simulink model "sampleModel1920"  (R2023a)
settings: Solver=VariableStepAuto  StartTime=0.0  StopTime=10.0  RelTol=1e-3
libraries: hdlsllib x4, simulink x2
settings Model: Creator=user1  LastModifiedBy=user1

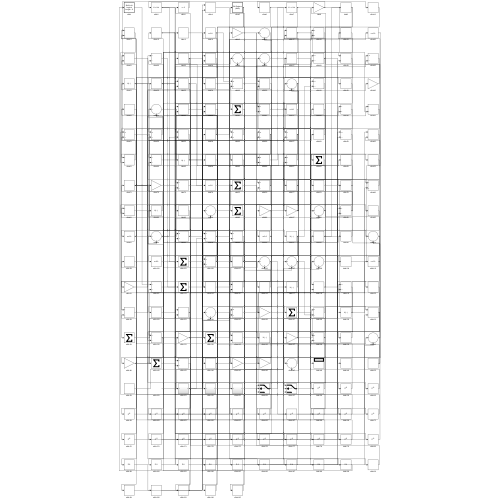
[thumbnail: Simulink's stored preview of the top-level diagram]
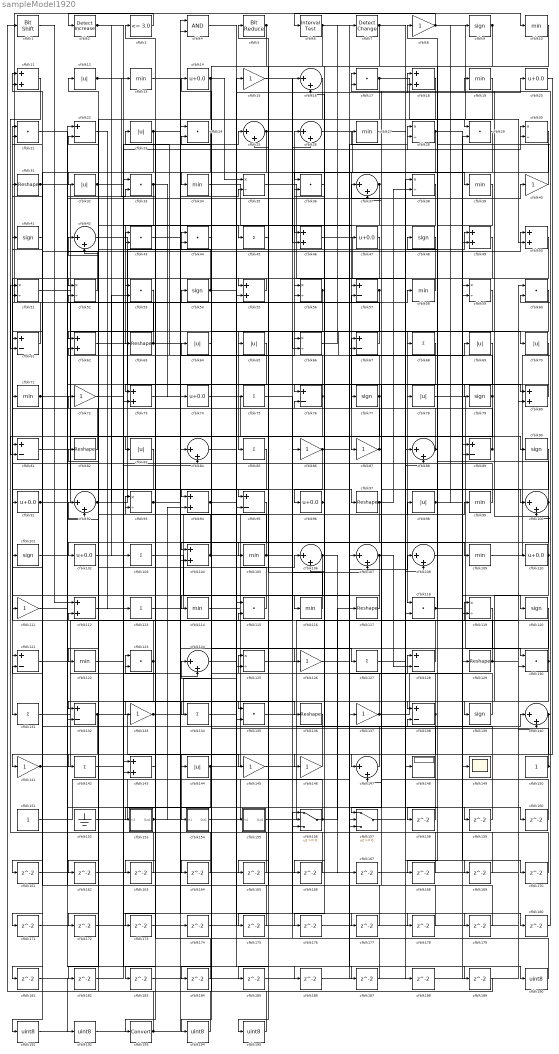
== system sampleModel1920 ==
  cfblk1 : hdlsllib/Logic and Bit Operations/Bit Shift  mode=Shift Left Logical  N=0
  cfblk{10,13,19,27,34,39,58,71,99,105,109,114,116,122} (14 alike) : MinMax
  cfblk{16,25..26,37,42,84,88,92,100,106..108,124,140,147} (15 alike) : Sum  Inputs=|++
  cfblk{9,41,48,54,77,79,90,101,120,139} (10 alike) : Signum
  cfblk{14,20,47,74,91,96,102,110} (8 alike) : Bias  Bias=0.0  SaturateOnIntegerOverflow=off
  cfblk{45,68,75,85,103,113,127,131,134,142} (10 alike) : Sum  Inputs=+
  cfblk{11,18,46,49..50,55,62,73,80,94,104,112,143} (13 alike) : Sum
  cfblk{8,15,40,72,86..87,111,126,133,137,141,145..146} (13 alike) : Gain
  cfblk{17,21,24,29,33,36,43..44,53,60,115,118,123,130,135} (15 alike) : DotProduct  OutDataTypeStr=Inherit: Inherit via internal rule
  cfblk{31,63,82,97,117,129,136} (7 alike) : Reshape
  cfblk{28,30,35,38,51..52,56,59,66,93,119,125} (12 alike) : Product  Inputs=*/  RndMeth=Zero  SaturateOnIntegerOverflow=on
  cfblk{12,23,32,64..65,69..70,78,83,98,144} (11 alike) : Abs  SaturateOnIntegerOverflow=off
  cfblk{22,57,61,67,76,81,89,95,121,128,132,138} (12 alike) : Sum  Inputs=+-
  cfblk148 : Display
  cfblk149 : Scope
  cfblk150 : Constant  SampleTime=-1
  cfblk151 : Constant  SampleTime=-1
  cfblk152 : Ground
  cfblk153 : Subsystem
      settings: LibrarySourceBlock=|
      | hdlsllib/Ports &
      | Subsystems/Subsystem
  cfblk154 : Subsystem
      settings: LibrarySourceBlock=|
      | hdlsllib/Ports &
      | Subsystems/Subsystem
  cfblk155 : Subsystem
      settings: LibrarySourceBlock=|
      | hdlsllib/Ports &
      | Subsystems/Subsystem
  cfblk156 : Switch  SaturateOnIntegerOverflow=off  InputSameDT=off
  cfblk157 : Switch  SaturateOnIntegerOverflow=off  InputSameDT=off
  cfblk{158..189} (32 alike) : Delay  SampleTime=1
  cfblk{190..192,194..195} (5 alike) : DataTypeConversion  OutDataTypeStr=uint8  SaturateOnIntegerOverflow=off  RndMeth=Floor
  cfblk193 : DataTypeConversion  SaturateOnIntegerOverflow=off  RndMeth=Floor
  cfblk2 : simulink/Logic and Bit Operations/Detect Increase  vinit=0.0  OutDataTypeStr=boolean
      settings: LibrarySourceBlock=|
      | hdlsllib/Logic and Bit
      | Operations/Detect
      | Increase
  cfblk3 : hdlsllib/Logic and Bit Operations/Compare To Constant  relop=<=  const=3.0  OutDataTypeStr=boolean
  cfblk4 : Logic  AllPortsSameDT=off  OutDataTypeStr=boolean
  cfblk5 : hdlsllib/Logic and Bit Operations/Bit Reduce  mode=AND
  cfblk6 : hdlsllib/Logic and Bit Operations/Interval Test  IntervalClosedRight=on  uplimit=0.5  IntervalClosedLeft=on  lowlimit=-0.5  OutDataTypeStr=boolean
  cfblk7 : simulink/Logic and Bit Operations/Detect Change  vinit=0  OutDataTypeStr=boolean
      settings: LibrarySourceBlock=|
      | hdlsllib/Logic and Bit
      | Operations/Detect
      | Change
  wires:
  cfblk66/1 -> cfblk7/1
  cfblk86/1 -> cfblk96/1, cfblk28/2
  cfblk1/1 -> cfblk112/1
  cfblk68/1 -> cfblk118/1
  cfblk33/1 -> cfblk74/1, cfblk52/1
  cfblk2/1 -> cfblk103/1, cfblk66/2, cfblk177/1
  cfblk78/1 -> cfblk130/1
  cfblk60/1 -> cfblk23/1
  cfblk136/1 -> cfblk154/1(In1)
  cfblk22/1 -> cfblk113/1
  cfblk56/1 -> cfblk85/1, cfblk135/1
  cfblk109/1 -> cfblk17/1
  cfblk128/1 -> cfblk13/1
  cfblk134/1 -> cfblk15/1
  cfblk20/1 -> cfblk147/1
  cfblk59/1 -> cfblk78/1
  cfblk62/1 -> cfblk49/1
  cfblk42/1 -> cfblk76/1
  cfblk30/1 -> cfblk87/1
  cfblk144/1 -> cfblk106/1, cfblk173/1
  cfblk58/1 -> cfblk57/1
  cfblk150/1 -> cfblk44/1, cfblk100/2
  cfblk153/1(Out1) -> cfblk99/1, cfblk94/2, cfblk57/2
  cfblk113/1 -> cfblk98/1
  cfblk129/1 -> cfblk110/1, cfblk93/1
  cfblk132/1 -> cfblk145/1, cfblk181/1
  cfblk115/1 -> cfblk12/1
  cfblk84/1 -> cfblk109/1
  cfblk92/1 -> cfblk58/1, cfblk53/2
  cfblk61/1 -> cfblk10/1
  cfblk3/1 -> cfblk2/1
  cfblk117/1 -> cfblk116/1
  cfblk12/1 -> cfblk45/1, cfblk97/1
  cfblk45/1 -> cfblk95/1
  cfblk49/1 -> cfblk131/1
  cfblk6/1 -> cfblk79/1, cfblk34/1
  cfblk77/1 -> cfblk26/1, cfblk156/3
  cfblk47/1 -> cfblk55/1
  cfblk87/1 -> cfblk21/1, cfblk27/1, cfblk37/2
  cfblk131/1 -> cfblk123/1
  cfblk155/1(Out1) -> cfblk140/1
  cfblk118/1 -> cfblk18/1, cfblk120/1
  cfblk122/1 -> cfblk25/1
  cfblk106/1 -> cfblk134/1, cfblk167/1
  cfblk46/1 -> cfblk88/1
  cfblk107/1 -> cfblk121/1, cfblk128/2
  cfblk111/1 -> cfblk50/1
  cfblk36/1 -> cfblk106/2
  cfblk91/1 -> cfblk54/1, cfblk11/2
  cfblk141/1 -> cfblk86/1, cfblk66/1
  cfblk31/1 -> cfblk70/1, cfblk186/1
  cfblk93/1 -> cfblk3/1, cfblk28/1
  cfblk96/1 -> cfblk36/2, cfblk166/1
  cfblk24/1 -> cfblk193/1
  cfblk54/1 -> cfblk22/2, cfblk20/1
  cfblk105/1 -> cfblk16/1, cfblk107/2, cfblk82/1, cfblk180/1
  cfblk135/1 -> cfblk38/1
  cfblk76/1 -> cfblk5/1, cfblk94/1, cfblk62/2
  cfblk81/1 -> cfblk90/1
  cfblk146/1 -> cfblk141/1
  cfblk52/1 -> cfblk11/1
  cfblk15/1 -> cfblk47/1
  cfblk37/1 -> cfblk63/1, cfblk157/2
  cfblk102/1 -> cfblk143/1
  cfblk108/1 -> cfblk149/1
  cfblk139/1 -> cfblk44/2
  cfblk55/1 -> cfblk53/1
  cfblk38/1 -> cfblk83/1
  cfblk90/1 -> cfblk147/2
  cfblk123/1 -> cfblk71/1, cfblk132/2
  cfblk14/1 -> cfblk32/1, cfblk35/1
  cfblk48/1 -> cfblk118/2
  cfblk16/1 -> cfblk55/2
  cfblk69/1 -> cfblk157/1
  cfblk156/1 -> cfblk125/1, cfblk117/1
  cfblk17/1 -> cfblk29/1, cfblk62/1
  cfblk140/1 -> cfblk60/2, cfblk191/1
  cfblk99/1 -> cfblk81/1
  cfblk43/1 -> cfblk127/1
  cfblk18/1 -> cfblk102/1
  cfblk10/1 -> cfblk68/1
  cfblk94/1 -> cfblk18/2, cfblk184/1
  cfblk114/1 -> cfblk49/2
  cfblk152/1 -> cfblk128/1
  cfblk80/1 -> cfblk73/1
  cfblk137/1 -> cfblk59/1, cfblk43/1
  cfblk95/1 -> cfblk122/1
  cfblk138/1 -> cfblk37/1, cfblk142/1
  cfblk119/1 -> cfblk138/1
  cfblk44/1 -> cfblk104/1
  cfblk133/1 -> cfblk75/1, cfblk159/1
  cfblk89/1 -> cfblk67/1, cfblk48/1
  cfblk79/1 -> cfblk81/2, cfblk16/2
  cfblk121/1 -> cfblk33/2
  cfblk97/1 -> cfblk38/2, cfblk182/1, cfblk183/1
  cfblk23/1 -> cfblk133/1, cfblk111/1, cfblk105/1
  cfblk88/1 -> cfblk43/2, cfblk168/1
  cfblk25/1 -> cfblk39/1, cfblk132/1
  cfblk145/1 -> cfblk60/1
  cfblk41/1 -> cfblk61/1
  cfblk51/1 -> cfblk115/1
  cfblk11/1 -> cfblk61/2
  cfblk29/1 -> cfblk91/1
  cfblk73/1 -> cfblk77/1
  cfblk5/1 -> cfblk114/1, cfblk135/2
  cfblk130/1 -> cfblk143/2, cfblk146/1, cfblk101/1, cfblk165/1
  cfblk9/1 -> cfblk36/1, cfblk126/1
  cfblk116/1 -> cfblk25/2
  cfblk101/1 -> cfblk56/1
  cfblk71/1 -> cfblk124/2, cfblk41/1, cfblk92/2, cfblk40/1, cfblk157/3
  cfblk67/1 -> cfblk42/2
  cfblk103/1 -> cfblk137/1
  cfblk100/1 -> cfblk64/1, cfblk175/1, cfblk176/1
  cfblk57/1 -> cfblk56/2, cfblk144/1
  cfblk154/1(Out1) -> cfblk108/1
  cfblk26/1 -> cfblk108/2
  cfblk104/1 -> cfblk26/2, cfblk52/2
  cfblk40/1 -> cfblk8/1
  cfblk35/1 -> cfblk148/1
  cfblk74/1 -> cfblk129/1
  cfblk8/1 -> cfblk50/2, cfblk6/1
  cfblk110/1 -> cfblk19/1, cfblk139/1
  cfblk34/1 -> cfblk46/1
  cfblk19/1 -> cfblk104/2
  cfblk28/1 -> cfblk46/2, cfblk170/1
  cfblk157/1 -> cfblk88/2
  cfblk151/1 -> cfblk69/1
  cfblk7/1 -> cfblk100/1, cfblk195/1
  cfblk98/1 -> cfblk89/2, cfblk9/1
  cfblk32/1 -> cfblk136/1, cfblk30/1
  cfblk82/1 -> cfblk72/1
  cfblk124/1 -> cfblk155/1(In1)
  cfblk125/1 -> cfblk119/1
  cfblk65/1 -> cfblk153/1(In1)
  cfblk21/1 -> cfblk80/1
  cfblk112/1 -> cfblk84/2
  cfblk147/1 -> cfblk51/2
  cfblk63/1 -> cfblk65/1, cfblk31/1, cfblk35/2
  cfblk39/1 -> cfblk158/1
  cfblk158/1 -> cfblk76/2
  cfblk159/1 -> cfblk138/2
  cfblk75/1 -> cfblk160/1
  cfblk160/1 -> cfblk112/2
  cfblk50/1 -> cfblk161/1
  cfblk161/1 -> cfblk95/2
  cfblk53/1 -> cfblk162/1
  cfblk162/1 -> cfblk29/2
  cfblk143/1 -> cfblk163/1
  cfblk163/1 -> cfblk33/1
  cfblk120/1 -> cfblk164/1
  cfblk164/1 -> cfblk51/1
  cfblk165/1 -> cfblk121/2
  cfblk166/1 -> cfblk42/1
  cfblk167/1 -> cfblk140/2
  cfblk168/1 -> cfblk156/1
  cfblk127/1 -> cfblk169/1
  cfblk169/1 -> cfblk124/1
  cfblk170/1 -> cfblk93/2
  cfblk85/1 -> cfblk171/1
  cfblk171/1 -> cfblk84/1
  cfblk83/1 -> cfblk172/1
  cfblk172/1 -> cfblk107/1
  cfblk173/1 -> cfblk125/2
  cfblk174/1 -> cfblk59/2
  cfblk175/1 -> cfblk21/2
  cfblk176/1 -> cfblk130/2
  cfblk177/1 -> cfblk115/2
  cfblk13/1 -> cfblk178/1
  cfblk178/1 -> cfblk17/2
  cfblk72/1 -> cfblk179/1
  cfblk179/1 -> cfblk22/1
  cfblk180/1 -> cfblk30/2
  cfblk182/1 -> cfblk73/2
  cfblk183/1 -> cfblk80/2
  cfblk184/1 -> cfblk123/2
  cfblk70/1 -> cfblk185/1
  cfblk185/1 -> cfblk67/2
  cfblk186/1 -> cfblk119/2
  cfblk142/1 -> cfblk187/1
  cfblk187/1 -> cfblk156/2
  cfblk27/1 -> cfblk188/1
  cfblk188/1 -> cfblk89/1
  cfblk126/1 -> cfblk189/1
  cfblk189/1 -> cfblk1/1
  cfblk4/1 -> cfblk190/1
  cfblk190/1 -> cfblk14/1
  cfblk191/1 -> cfblk4/1
  cfblk181/1 -> cfblk192/1
  cfblk192/1 -> cfblk4/2
  cfblk193/1 -> cfblk174/1, cfblk92/1
  cfblk64/1 -> cfblk194/1
  cfblk194/1 -> cfblk24/1
  cfblk195/1 -> cfblk24/2

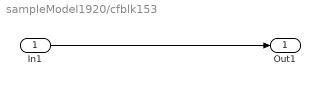
== system sampleModel1920/cfblk153 ==
  In1 : Inport
  Out1 : Outport
  wires:
  In1/1 -> Out1/1

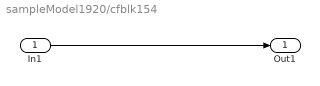
== system sampleModel1920/cfblk154 ==
  In1 : Inport
  Out1 : Outport
  wires:
  In1/1 -> Out1/1

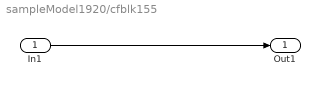
== system sampleModel1920/cfblk155 ==
  In1 : Inport
  Out1 : Outport
  wires:
  In1/1 -> Out1/1
